simulink model "MPC_FL_CBFcontroller"  (R2026a)
settings: Solver=VariableStepAuto  StopTime=120
PreLoadFcn:
  | % Define variants
  | VSS_PATH_CTRL_PURE_PURSUIT=Simulink.Variant('VSS_PATH_CTRL_MODE==1');
  | VSS_PATH_CTRL_REAR_WHEEL=Simulink.Variant('VSS_PATH_CTRL_MODE==2');
  | % Select default variant
  | VSS_PATH_CTRL_MODE =1;
  | 
  | 
  | % Longitudinal PID
  | LongitudinalPID.Kp = 20;
  | LongitudinalPID.Ki = 0;
  | LongitudinalPID.Kd = 0;
  | LongitudinalPID.N = 100;
  | LongitudinalPID.MaxAccel = 80;
  | LongitudinalPID.SampleTime = 0.01;
  | 
  | % Steering PID
  | SteeringPID.Kp = 60;
  | SteeringPID.Ki = 0;
  | SteeringPID.Kd = 5;
  | SteeringPID.N = 10;
  | SteeringPID.MaxSpeed =  10;
  | SteeringPID.MinSpeed = -10;
  | SteeringPID.SampleTime = 0.01;
  | 
  | 
  | 
  | setSMVehicleVisuParameters;
  | 
  | % Load planner commands
  | load('PlannerCmdTests.mat');
  | % Assign one for testing:
  | plannerCmd = plannerCmdFwd;
  | % plannerCmd  = plannerCmdFwdBwd;
  | 
  | % Bus structure definition
  | load('PlannerBusStruct.mat');
  | 
  | % Rear Wheel Controller Parameters
  | RW.k_e = 0.2;    % 0.1
  | RW.k_theta = 1;   % 0.75
  | RW.SampleTime =  0.1;
  | RW.GoalRadius = 0.3;
  | 
  | % Pure pursuit parameters
  | PP.DesiredLinearVel = 5;
  | PP.MaxAngularVel  = 10;
  | PP.LookaheadDist  = 1;
  | PP.Wheelbase = 4;
  | PP.GoalRadius = 0.1;
  | PP.SampleTime = 0.1;
  | PP.LongitudinalPID.Kp = 20;
  | PP.LongitudinalPID.Ki = 0;
  | PP.LongitudinalPID.Kd = 0;
  | PP.LongitudinalPID.N = 100;
  | PP.LongitudinalPID.MaxLongAccel =  80;
  | PP.LongitudinalPID.MinLongAccel = -80;
  | 
  | % Spline ref
  | splineRef = [ 0 0 0;[plannerCmd.PathMatrix(1:plannerCmd.PathLengths(1),1:2,1),0*ones(length(plannerCmd.PathMatrix(1:plannerCmd.PathLengths(1),1,1)),1)]];
values from neighbouring files (symbols this model uses):
  m = max(2, ceil(Lseg/ds))    [Trajectory.m]    (also in plot_nmpc_result.m = NaN)
  s = [0; cumsum(hypot(diff(xs),diff(ys)))]    [Trajectory.m]    (also in plot_parking_mpc.m = evalin('base',name); plot_result.m = out.(names{k}))
  trajMatrix = [tvec, xd, yd, thd, vd, wd]    [Trajectory.m]    (also in plot_parking_mpc.m = evalin('base','trajMatrix'); plot_result.m = evalin('base','trajMatrix'))
undefined symbols (not defined in the file or in its folder): DiscIntNeverNeededParam, smvv, X, Y, Z
libraries: sm_lib x527, sm_vehicle_slalom_lib x48, fl_lib x40, fl_ps_legacy_lib x28, nesl_utility x13
(part 15 of 15)

== system MPC_FL_CBFcontroller/Robot Bicycle Model/Visualizer/SM_Car_Visu/Vehicle7/Steering_Wheel/Logo/LStick3 ==
  Stick : sm_lib/Body Elements/Brick Solid  BrickDimensions=[smvv.steeringwheel.letterStick 0.001 0.001]  BrickDimensionsUnits=m  ExportEntireGeometry=off  InertiaType=PointMass  BasedOnType=Density  Density=1000  DensityUnits=kg/m^3  Mass=0.001  MassUnits=kg  CenterOfMass=[0 0 0]  CenterOfMassUnits=m  MomentsOfInertia=[1 1 1]  MomentsOfInertiaUnits=kg*m^2  ProductsOfInertia=[1 1 1]  ProductsOfInertiaUnits=kg*m^2  GraphicType=FromGeometry  MarkerShape=Sphere  MarkerSize=10  GraphicVisPropType=SimpleVisualProperties  GraphicDiffuseColor=smvv.steeringwheel.letterColor  GraphicOpacity=1.0  GraphicSpecularColor=[0.5 0.5 0.5 1.0]  GraphicAmbientColor=[0.15 0.15 0.15 1.0]  GraphicEmissiveColor=[0.0 0.0 0.0 1.0]  GraphicShininess=75  DoExposeReferenceFrame=on  SerializedFrames=<Frames/>
  X offset 1 : sm_lib/Frames and Transforms/Rigid Transform  RotationMethod=None  FollAlignAxisA=+X  BaseAlignAxisA=+Y  FollAlignAxisB=+Y  BaseAlignAxisB=+Z  RotationStandardAxis=+X  RotationAngle=0  RotationAngleUnits=deg  RotationArbitraryAxis=[0 0 1]  RotationSequenceAxes=FollowerAxes  RotationSequence=XYX  RotationSequenceAngles=[0 0 0]  RotationSequenceAnglesUnits=deg  RotationMatrix=[1 0 0; 0 1 0; 0 0 1]  Quaternion=[1 0 0 0]  TranslationMethod=StandardAxis  TranslationCartesianOffset=[0 0 0]  TranslationCartesianOffsetUnits=m  TranslationStandardAxis=-X  TranslationStandardOffset=0.5*smvv.steeringwheel.letterStick  TranslationStandardOffsetUnits=m  TranslationROffset=0  TranslationROffsetUnits=m  TranslationThetaOffset=0  TranslationThetaOffsetUnits=deg  TranslationZOffset=0  TranslationZOffsetUnits=m
  x offset 2 : sm_lib/Frames and Transforms/Rigid Transform  RotationMethod=None  FollAlignAxisA=+X  BaseAlignAxisA=+Y  FollAlignAxisB=+Y  BaseAlignAxisB=+Z  RotationStandardAxis=+X  RotationAngle=0  RotationAngleUnits=deg  RotationArbitraryAxis=[0 0 1]  RotationSequenceAxes=FollowerAxes  RotationSequence=XYX  RotationSequenceAngles=[0 0 0]  RotationSequenceAnglesUnits=deg  RotationMatrix=[1 0 0; 0 1 0; 0 0 1]  Quaternion=[1 0 0 0]  TranslationMethod=StandardAxis  TranslationCartesianOffset=[0 0 0]  TranslationCartesianOffsetUnits=m  TranslationStandardAxis=+X  TranslationStandardOffset=0.5*smvv.steeringwheel.letterStick  TranslationStandardOffsetUnits=m  TranslationROffset=0  TranslationROffsetUnits=m  TranslationThetaOffset=0  TranslationThetaOffsetUnits=deg  TranslationZOffset=0  TranslationZOffsetUnits=m
  Conn1 : PMIOPort  Side=Left
  Conn2 : PMIOPort  Port=2  Side=Right
  connections:
  X offset 1/RConn1 -- Conn1/RConn1
  x offset 2/RConn1 -- Conn2/RConn1
  x offset 2/LConn1 -- Stick/RConn1 -- X offset 1/LConn1

== system MPC_FL_CBFcontroller/Robot Bicycle Model/Visualizer/SM_Car_Visu/Vehicle7/Steering_Wheel/Logo/LStick4 ==
  Stick : sm_lib/Body Elements/Brick Solid  BrickDimensions=[smvv.steeringwheel.letterStick 0.001 0.001]  BrickDimensionsUnits=m  ExportEntireGeometry=off  InertiaType=PointMass  BasedOnType=Density  Density=1000  DensityUnits=kg/m^3  Mass=0.001  MassUnits=kg  CenterOfMass=[0 0 0]  CenterOfMassUnits=m  MomentsOfInertia=[1 1 1]  MomentsOfInertiaUnits=kg*m^2  ProductsOfInertia=[1 1 1]  ProductsOfInertiaUnits=kg*m^2  GraphicType=FromGeometry  MarkerShape=Sphere  MarkerSize=10  GraphicVisPropType=SimpleVisualProperties  GraphicDiffuseColor=smvv.steeringwheel.letterColor  GraphicOpacity=1.0  GraphicSpecularColor=[0.5 0.5 0.5 1.0]  GraphicAmbientColor=[0.15 0.15 0.15 1.0]  GraphicEmissiveColor=[0.0 0.0 0.0 1.0]  GraphicShininess=75  DoExposeReferenceFrame=on  SerializedFrames=<Frames/>
  X offset 1 : sm_lib/Frames and Transforms/Rigid Transform  RotationMethod=None  FollAlignAxisA=+X  BaseAlignAxisA=+Y  FollAlignAxisB=+Y  BaseAlignAxisB=+Z  RotationStandardAxis=+X  RotationAngle=0  RotationAngleUnits=deg  RotationArbitraryAxis=[0 0 1]  RotationSequenceAxes=FollowerAxes  RotationSequence=XYX  RotationSequenceAngles=[0 0 0]  RotationSequenceAnglesUnits=deg  RotationMatrix=[1 0 0; 0 1 0; 0 0 1]  Quaternion=[1 0 0 0]  TranslationMethod=StandardAxis  TranslationCartesianOffset=[0 0 0]  TranslationCartesianOffsetUnits=m  TranslationStandardAxis=-X  TranslationStandardOffset=0.5*smvv.steeringwheel.letterStick  TranslationStandardOffsetUnits=m  TranslationROffset=0  TranslationROffsetUnits=m  TranslationThetaOffset=0  TranslationThetaOffsetUnits=deg  TranslationZOffset=0  TranslationZOffsetUnits=m
  Conn1 : PMIOPort  Side=Left
  connections:
  Stick/RConn1 -- X offset 1/LConn1
  X offset 1/RConn1 -- Conn1/RConn1

== system MPC_FL_CBFcontroller/Robot Bicycle Model/Visualizer/SM_Car_Visu/Vehicle7/Steering_Wheel/Logo/LStick5 ==
  Stick : sm_lib/Body Elements/Brick Solid  BrickDimensions=[smvv.steeringwheel.letterStick 0.001 0.001]  BrickDimensionsUnits=m  ExportEntireGeometry=off  InertiaType=PointMass  BasedOnType=Density  Density=1000  DensityUnits=kg/m^3  Mass=0.001  MassUnits=kg  CenterOfMass=[0 0 0]  CenterOfMassUnits=m  MomentsOfInertia=[1 1 1]  MomentsOfInertiaUnits=kg*m^2  ProductsOfInertia=[1 1 1]  ProductsOfInertiaUnits=kg*m^2  GraphicType=FromGeometry  MarkerShape=Sphere  MarkerSize=10  GraphicVisPropType=SimpleVisualProperties  GraphicDiffuseColor=smvv.steeringwheel.letterColor  GraphicOpacity=1.0  GraphicSpecularColor=[0.5 0.5 0.5 1.0]  GraphicAmbientColor=[0.15 0.15 0.15 1.0]  GraphicEmissiveColor=[0.0 0.0 0.0 1.0]  GraphicShininess=75  DoExposeReferenceFrame=on  SerializedFrames=<Frames/>
  X offset 1 : sm_lib/Frames and Transforms/Rigid Transform  RotationMethod=None  FollAlignAxisA=+X  BaseAlignAxisA=+Y  FollAlignAxisB=+Y  BaseAlignAxisB=+Z  RotationStandardAxis=+X  RotationAngle=0  RotationAngleUnits=deg  RotationArbitraryAxis=[0 0 1]  RotationSequenceAxes=FollowerAxes  RotationSequence=XYX  RotationSequenceAngles=[0 0 0]  RotationSequenceAnglesUnits=deg  RotationMatrix=[1 0 0; 0 1 0; 0 0 1]  Quaternion=[1 0 0 0]  TranslationMethod=StandardAxis  TranslationCartesianOffset=[0 0 0]  TranslationCartesianOffsetUnits=m  TranslationStandardAxis=-X  TranslationStandardOffset=0.5*smvv.steeringwheel.letterStick  TranslationStandardOffsetUnits=m  TranslationROffset=0  TranslationROffsetUnits=m  TranslationThetaOffset=0  TranslationThetaOffsetUnits=deg  TranslationZOffset=0  TranslationZOffsetUnits=m
  x offset 2 : sm_lib/Frames and Transforms/Rigid Transform  RotationMethod=None  FollAlignAxisA=+X  BaseAlignAxisA=+Y  FollAlignAxisB=+Y  BaseAlignAxisB=+Z  RotationStandardAxis=+X  RotationAngle=0  RotationAngleUnits=deg  RotationArbitraryAxis=[0 0 1]  RotationSequenceAxes=FollowerAxes  RotationSequence=XYX  RotationSequenceAngles=[0 0 0]  RotationSequenceAnglesUnits=deg  RotationMatrix=[1 0 0; 0 1 0; 0 0 1]  Quaternion=[1 0 0 0]  TranslationMethod=StandardAxis  TranslationCartesianOffset=[0 0 0]  TranslationCartesianOffsetUnits=m  TranslationStandardAxis=+X  TranslationStandardOffset=0.5*smvv.steeringwheel.letterStick  TranslationStandardOffsetUnits=m  TranslationROffset=0  TranslationROffsetUnits=m  TranslationThetaOffset=0  TranslationThetaOffsetUnits=deg  TranslationZOffset=0  TranslationZOffsetUnits=m
  Conn1 : PMIOPort  Side=Left
  Conn2 : PMIOPort  Port=2  Side=Right
  connections:
  X offset 1/RConn1 -- Conn1/RConn1
  x offset 2/RConn1 -- Conn2/RConn1
  x offset 2/LConn1 -- Stick/RConn1 -- X offset 1/LConn1

== system MPC_FL_CBFcontroller/Robot Bicycle Model/Visualizer/SM_Car_Visu/Vehicle7/Steering_Wheel/Logo/LStick6 ==
  Stick : sm_lib/Body Elements/Brick Solid  BrickDimensions=[2*smvv.steeringwheel.letterStick 0.001 0.001]  BrickDimensionsUnits=m  ExportEntireGeometry=off  InertiaType=PointMass  BasedOnType=Density  Density=1000  DensityUnits=kg/m^3  Mass=0.001  MassUnits=kg  CenterOfMass=[0 0 0]  CenterOfMassUnits=m  MomentsOfInertia=[1 1 1]  MomentsOfInertiaUnits=kg*m^2  ProductsOfInertia=[1 1 1]  ProductsOfInertiaUnits=kg*m^2  GraphicType=FromGeometry  MarkerShape=Sphere  MarkerSize=10  GraphicVisPropType=SimpleVisualProperties  GraphicDiffuseColor=smvv.steeringwheel.letterColor  GraphicOpacity=1.0  GraphicSpecularColor=[0.5 0.5 0.5 1.0]  GraphicAmbientColor=[0.15 0.15 0.15 1.0]  GraphicEmissiveColor=[0.0 0.0 0.0 1.0]  GraphicShininess=75  DoExposeReferenceFrame=on  SerializedFrames=<Frames/>
  X offset 1 : sm_lib/Frames and Transforms/Rigid Transform  RotationMethod=None  FollAlignAxisA=+X  BaseAlignAxisA=+Y  FollAlignAxisB=+Y  BaseAlignAxisB=+Z  RotationStandardAxis=+X  RotationAngle=0  RotationAngleUnits=deg  RotationArbitraryAxis=[0 0 1]  RotationSequenceAxes=FollowerAxes  RotationSequence=XYX  RotationSequenceAngles=[0 0 0]  RotationSequenceAnglesUnits=deg  RotationMatrix=[1 0 0; 0 1 0; 0 0 1]  Quaternion=[1 0 0 0]  TranslationMethod=StandardAxis  TranslationCartesianOffset=[0 0 0]  TranslationCartesianOffsetUnits=m  TranslationStandardAxis=-X  TranslationStandardOffset=smvv.steeringwheel.letterStick  TranslationStandardOffsetUnits=m  TranslationROffset=0  TranslationROffsetUnits=m  TranslationThetaOffset=0  TranslationThetaOffsetUnits=deg  TranslationZOffset=0  TranslationZOffsetUnits=m
  x offset 2 : sm_lib/Frames and Transforms/Rigid Transform  RotationMethod=None  FollAlignAxisA=+X  BaseAlignAxisA=+Y  FollAlignAxisB=+Y  BaseAlignAxisB=+Z  RotationStandardAxis=+X  RotationAngle=0  RotationAngleUnits=deg  RotationArbitraryAxis=[0 0 1]  RotationSequenceAxes=FollowerAxes  RotationSequence=XYX  RotationSequenceAngles=[0 0 0]  RotationSequenceAnglesUnits=deg  RotationMatrix=[1 0 0; 0 1 0; 0 0 1]  Quaternion=[1 0 0 0]  TranslationMethod=StandardAxis  TranslationCartesianOffset=[0 0 0]  TranslationCartesianOffsetUnits=m  TranslationStandardAxis=+X  TranslationStandardOffset=smvv.steeringwheel.letterStick  TranslationStandardOffsetUnits=m  TranslationROffset=0  TranslationROffsetUnits=m  TranslationThetaOffset=0  TranslationThetaOffsetUnits=deg  TranslationZOffset=0  TranslationZOffsetUnits=m
  Conn1 : PMIOPort  Side=Left
  Conn2 : PMIOPort  Port=2  Side=Right
  connections:
  X offset 1/LConn1 -- Stick/RConn1 -- x offset 2/LConn1
  x offset 2/RConn1 -- Conn2/RConn1
  X offset 1/RConn1 -- Conn1/RConn1

== system MPC_FL_CBFcontroller/Robot Bicycle Model/Visualizer/SM_Car_Visu/Vehicle7/Steering_Wheel/Logo/LStick7 ==
  Stick : sm_lib/Body Elements/Brick Solid  BrickDimensions=[smvv.steeringwheel.letterStick 0.001 0.001]  BrickDimensionsUnits=m  ExportEntireGeometry=off  InertiaType=PointMass  BasedOnType=Density  Density=1000  DensityUnits=kg/m^3  Mass=0.001  MassUnits=kg  CenterOfMass=[0 0 0]  CenterOfMassUnits=m  MomentsOfInertia=[1 1 1]  MomentsOfInertiaUnits=kg*m^2  ProductsOfInertia=[1 1 1]  ProductsOfInertiaUnits=kg*m^2  GraphicType=FromGeometry  MarkerShape=Sphere  MarkerSize=10  GraphicVisPropType=SimpleVisualProperties  GraphicDiffuseColor=smvv.steeringwheel.letterColor  GraphicOpacity=1.0  GraphicSpecularColor=[0.5 0.5 0.5 1.0]  GraphicAmbientColor=[0.15 0.15 0.15 1.0]  GraphicEmissiveColor=[0.0 0.0 0.0 1.0]  GraphicShininess=75  DoExposeReferenceFrame=on  SerializedFrames=<Frames/>
  X offset 1 : sm_lib/Frames and Transforms/Rigid Transform  RotationMethod=None  FollAlignAxisA=+X  BaseAlignAxisA=+Y  FollAlignAxisB=+Y  BaseAlignAxisB=+Z  RotationStandardAxis=+X  RotationAngle=0  RotationAngleUnits=deg  RotationArbitraryAxis=[0 0 1]  RotationSequenceAxes=FollowerAxes  RotationSequence=XYX  RotationSequenceAngles=[0 0 0]  RotationSequenceAnglesUnits=deg  RotationMatrix=[1 0 0; 0 1 0; 0 0 1]  Quaternion=[1 0 0 0]  TranslationMethod=StandardAxis  TranslationCartesianOffset=[0 0 0]  TranslationCartesianOffsetUnits=m  TranslationStandardAxis=-X  TranslationStandardOffset=0.5*smvv.steeringwheel.letterStick  TranslationStandardOffsetUnits=m  TranslationROffset=0  TranslationROffsetUnits=m  TranslationThetaOffset=0  TranslationThetaOffsetUnits=deg  TranslationZOffset=0  TranslationZOffsetUnits=m
  Conn1 : PMIOPort  Side=Left
  connections:
  X offset 1/RConn1 -- Conn1/RConn1
  Stick/RConn1 -- X offset 1/LConn1

== matlab function MPC_FL_CBFcontroller/MATLAB Function1 ==
  data: pose input; v_out output; u1_cmd input; u2_cmd input; delta_out output; h_min_out output; qp_status output; h_red_out output; h_pink_out output; h_obs3_out output
function [v_out, delta_out, h_min_out, qp_status, ...
          h_red_out, h_pink_out, h_obs3_out] = ...
    fl_cbf_inner_filter_u1u2_reverse(pose, u1_cmd, u2_cmd)
% Fast feedback-linearization + CBF safety filter for the reverse-phase outer.
%
% Inputs u1_cmd and u2_cmd are the virtual velocity of the point
%   P = [x;y] + ell*[cos(theta);sin(theta)].
% This block converts them to q = [v; v*tan(delta)] and projects q into
% the CBF-safe and actuator-limited set.

coder.extrinsic('quadprog');
coder.extrinsic('optimoptions');

%% Parameters
% IMPORTANT: set this equal to the sample time of this MATLAB Function
% block. For a 100 Hz inner loop use 0.01; for 50 Hz use 0.02.
Ts = 0.01;

L        = 3.0;
ell      = L;
vMin     = -2.5;
vMax     =  3.0;
dMax     = 60*pi/180;
tanDMax  = tan(dMax);
aMax     = 3.0;
dRate    = 0.60;
gammaCBF = 0.30;

% Obstacle circles: [cx, cy, inflated radius].
obs = [53.5, 21.0, 3.64;   % red, rear  (unchanged)
    56.5, 21.0, 3.64;   % red, front (unchanged)
    37.5, 21.0, 3.64;   % pink, rear  ← FIX: was 38.5, should be 37.5
    40.5, 21.0, 3.64;   % pink, front (correct)
    26.6, 17.0, 3.24];  % obstacle 3  (unchanged)

nObs = 5;

%% Persistent actuator state and gear hysteresis
persistent prevV prevDelta gear

if isempty(prevV) || isempty(prevDelta) || isempty(gear)
    prevV     = 0.0;
    prevDelta = 0.0;
    gear      = 1.0;
end

pose = double(pose(:));
pose = pose(1:3);
pose(3) = atan2(sin(pose(3)),cos(pose(3)));

uRef = [double(u1_cmd);double(u2_cmd)];

th = pose(3);
eTheta = [cos(th);sin(th)];
ePerp  = [-sin(th);cos(th)];

% P_dot = eTheta*v + (ell/L)*ePerp*(v*tan(delta)).
% Therefore:
%   v          = eTheta.'*uRef
%   v*tan(del) = (L/ell)*ePerp.'*uRef
vNom  = eTheta.'*uRef;
q2Nom = (L/ell)*(ePerp.'*uRef);
vNom  = max(vMin,min(vMax,vNom));

% Gear hysteresis prevents rapid switching between forward and reverse
% steering cones when the planned longitudinal velocity crosses zero.
if gear >= 0.0
    if vNom < -0.15
        gear = -1.0;
    end
else
    if vNom > 0.15
        gear = 1.0;
    end
end

if abs(vNom) <= 0.15 && abs(prevV) > 0.20
    gear = sign(prevV);
end

%% Current barrier diagnostics
hRedOut = minimumBarrierAgainstSet(pose,obs(1:2,:),L);
hPinkOut = minimumBarrierAgainstSet(pose,obs(3:4,:),L);
hObs3Out = minimumBarrierAgainstSet(pose,obs(5:5,:),L);

h_red_out  = hRedOut;
h_pink_out = hPinkOut;
h_obs3_out = hObs3Out;
h_min_out  = min(hRedOut,min(hPinkOut,hObs3Out));

%% Nominal auxiliary input obtained from feedback linearization
qNom = [vNom;q2Nom];

% Penalize changes in velocity more than changes in the auxiliary steering
% variable. The exact steering wheel is recovered after the QP.
wV = 8.0;
wQ = 2.0;

H = diag([2.0*wV,2.0*wQ]);
f = [-2.0*wV*qNom(1);
     -2.0*wQ*qNom(2)];

% Suppress repeated solver messages in the Simulation Diagnostics window.
qpOptions = optimoptions('quadprog', ...
    'Algorithm','interior-point-convex','Display','off');

%% Bounds and actuator-rate limits
dvMax = aMax*Ts;
ddMax = dRate*Ts;

q2Prev = prevV*tan(prevDelta);

% This box is a conservative linear approximation of steering-rate
% limiting in q-space.
dq2Max = abs(prevV)*ddMax + dvMax*tanDMax + 0.02;

lb = [max(vMin,prevV-dvMax);
      max(-vMax*tanDMax,q2Prev-dq2Max)];

ub = [min(vMax,prevV+dvMax);
      min( vMax*tanDMax,q2Prev+dq2Max)];

%% Try the selected gear cone first, then the opposite cone if necessary
qSol       = [0.0;0.0];
exitStatus = -100.0;
solved     = false;
usedGear   = gear;

for attempt = 1:2
    if attempt == 1
        gearTry = gear;
    else
        gearTry = -gear;
    end

    Aineq = zeros(2*nObs+2,2);
    bineq = zeros(2*nObs+2,1);
    row = 0;

    % Exact sufficient linear DCBF constraints for both ego circles.
    for j = 1:nObs
        cx = obs(j,1);
        cy = obs(j,2);
        rr = obs(j,3);

        [hRear,aRear] = rearCbfRow(pose,cx,cy,rr,Ts);
        row = row+1;
        Aineq(row,:) = aRear.';
        bineq(row)   = gammaCBF*hRear;

        [hFront,aFront] = frontCbfRow(pose,cx,cy,rr,Ts,L);
        row = row+1;
        Aineq(row,:) = aFront.';
        bineq(row)   = gammaCBF*hFront;
    end

    % Steering cone. Because q2=v*tan(delta), the feasible steering cone
    % depends on the direction of motion.
    if gearTry >= 0.0
        % Forward: |q2| <= tan(dMax)*q1. This also enforces q1 >= 0.
        row = row+1;
        Aineq(row,:) = [-tanDMax,  1.0];
        bineq(row)   = 0.0;

        row = row+1;
        Aineq(row,:) = [-tanDMax, -1.0];
        bineq(row)   = 0.0;
    else
        % Reverse: tan(dMax)*q1 <= q2 <= -tan(dMax)*q1.
        % This also enforces q1 <= 0.
        row = row+1;
        Aineq(row,:) = [tanDMax,  1.0];
        bineq(row)   = 0.0;

        row = row+1;
        Aineq(row,:) = [tanDMax, -1.0];
        bineq(row)   = 0.0;
    end

    % quadprog returns an empty q when it declares the QP infeasible.
    % Keep the raw output variable-size and copy only after checking its
    % length, preventing a 2x1 versus 0x0 runtime mismatch.
    qTryRaw = zeros(0,1);
    coder.varsize('qTryRaw',[2 1],[true false]);
    exitTry = 0.0;

    [qTryRaw,~,exitTry] = quadprog( ...
        H,f,Aineq,bineq,[],[],lb,ub,[],qpOptions);

    qTry = zeros(2,1);
    qTryOK = false;

    if exitTry > 0 && size(qTryRaw,1) == 2
        qTry(:) = qTryRaw(1:2);
        qTryOK = true;

        if ~isfinite(qTry(1)) || ~isfinite(qTry(2))
            qTryOK = false;
        end
    end

    if qTryOK
        qSol       = qTry;
        exitStatus = exitTry;
        solved     = true;
        usedGear   = gearTry;
        break;
    end
end

%% Convert auxiliary input to actuator commands
if solved
    vOut = qSol(1);

    if abs(vOut) < 1e-4
        vOut     = 0.0;
        deltaOut = prevDelta;
    else
        deltaOut = atan(qSol(2)/vOut);
    end

    vOut     = max(vMin,min(vMax,vOut));
    deltaOut = max(-dMax,min(dMax,deltaOut));

    % Keep the persistent cone consistent with the successful QP cone.
    gear = usedGear;
else
    % If both cones are infeasible, stop. If the current state is safe,
    % zero velocity keeps the one-step state inside the safe set.
    vOut       = 0.0;
    deltaOut   = prevDelta;
    exitStatus = -10.0;
end

v_out     = vOut;
delta_out = deltaOut;
qp_status = exitStatus;

prevV     = v_out;
prevDelta = delta_out;

end

%% -----------------------------------------------------------------------
function hMin = minimumBarrierAgainstSet(x,obsSet,L)

nLocal = size(obsSet,1);
hMin = 1.0e12;

for j = 1:nLocal
    cx = obsSet(j,1);
    cy = obsSet(j,2);
    rr = obsSet(j,3);

    hRear = rearBarrier(x,cx,cy,rr);
    hFront = frontBarrier(x,cx,cy,rr,L);
    hBoth = min(hRear,hFront);

    if hBoth < hMin
        hMin = hBoth;
    end
end

end

%% -----------------------------------------------------------------------
function h = rearBarrier(x,cx,cy,r)

dx = x(1)-cx;
dy = x(2)-cy;
h  = dx*dx+dy*dy-r*r;

end

%% -----------------------------------------------------------------------
function h = frontBarrier(x,cx,cy,r,L)

th = x(3);
px = x(1)+L*cos(th);
py = x(2)+L*sin(th);

dx = px-cx;
dy = py-cy;
h  = dx*dx+dy*dy-r*r;

end

%% -----------------------------------------------------------------------
function [h,a] = rearCbfRow(x,cx,cy,r,Ts)
% Rear ego center moves as p_next = p + Ts*e*q1.
% h_next = h + 2*d'*G*q + ||G*q||^2, so
% 2*d'*G*q >= -gamma*h is sufficient for h_next >= (1-gamma)*h.

th = x(3);
e = [cos(th);sin(th)];

d = [x(1)-cx;
     x(2)-cy];

h = d.'*d-r*r;

G = [Ts*e, zeros(2,1)];

% We need 2*d'*G*q >= -gamma*h, i.e. -2*d'*G*q <= gamma*h.
a = -2.0*(d.'*G).';

end

%% -----------------------------------------------------------------------
function [h,a] = frontCbfRow(x,cx,cy,r,Ts,L)
% Front ego center moves as
% p_next = p + Ts*e*q1 + Ts*e_perp*q2,
% where q2 = v*tan(delta).

th = x(3);
e     = [cos(th);sin(th)];
ePerp = [-sin(th);cos(th)];

px = x(1)+L*cos(th);
py = x(2)+L*sin(th);

d = [px-cx;
     py-cy];

h = d.'*d-r*r;

G = Ts*[e,ePerp];

a = -2.0*(d.'*G).';

end

== matlab function MPC_FL_CBFcontroller/MATLAB Function ==
  data: pose input; trajectory input; u1_cmd output; t input; u2_cmd output; P_pred_out output; qp_status output; scp_passes_out output; mode_out output
function [u1_cmd, u2_cmd, P_pred_out, qp_status, scp_passes_out, mode_out] = ...
    mpc_outer_linear_cbf_reverse(pose, trajectory, t)
% Updated outer MPC-CBF for the feedback-linearized vehicle point P.
%
% Inputs:
%   pose       = [x_rear; y_rear; theta]
%   trajectory = [t, x_rear, y_rear, theta, v, kappa]
%   t          = current simulation time
%
% Outputs:
%   u1_cmd,u2_cmd  virtual velocity of the feedback-linearized point P
%   P_pred_out     2 x (Np+1) predicted positions of P
%   qp_status      status of the last successful QP
%   scp_passes_out number of successful SCP passes
%   mode_out       1=TRACK, 2=AVOID, 3=REJOIN, 4=STOP AT S-START,
%                    5=REVERSE-S, 6=PARKED
%
% Important:
%   This version preserves the u1/u2 feedback-linearized architecture.
%   The inner block must convert [u1;u2] to [v;delta] using the same
%   feedback-linearization distance ell = L.

coder.extrinsic('quadprog');
coder.extrinsic('optimoptions');

%% User parameters
Ts   = 0.20;
Np   = 5;
nSCP = 3;

L   = 3.0;
ell = L;

uMax = 3.0;

Q     = 20.0*eye(2);
Qf    = 80.0*eye(2);
R     = 0.40*eye(2);
rhoDu = 1.20;

gammaCBF = 0.3;
scpTrust = 1.25;

%% Vehicle and obstacle parameters
rVeh        = 1.6;
carHalfSpace = 1.5;
marginOuter = 0.4 + 0.05*0.8;
marginInner = marginOuter;

% Conservative single-circle model around the feedback-linearized point P.
% For either parked car:
%   parked-car envelope = 1.5 + 1.6 = 3.1 m
%   ego envelope around P = ell + 1.6 = 3.1 m
%   total separation      = 3.1 + 3.1 + 0.44 = 6.64 m
% Reduced outer planning radius. The inner two-circle CBF remains the
% exact hard safety layer, so the outer single circle need not carry the
% full midpoint-envelope inflation.
rOuterCar = 4.20;

% Obstacle 3 has physical radius 1.2 m.
rObs3   = 1.2;
% Slightly larger than the exact inner separation of 3.24 m, but much
% less conservative than the full midpoint-envelope value of 4.74 m.
rOuter3 = 3.30;

% Exact two-ego-circle separation used for mode-exit diagnostics.
rPair3 = rObs3+rVeh+marginInner;

% [cx, cy, outer-MPC radius]
obs = [55.0, 21.0, rOuterCar;   % red parked car
       39.0, 21.0, rOuterCar;   % pink parked car
       26.6, 17.0, rOuter3];    % obstacle 3

nObs = 3;

xObs3 = obs(3,1);
yObs3 = obs(3,2);

% Rear-axle progress gates. The corresponding P gates are obtained by
% shifting ell forward because the gate heading is approximately zero.
gateRear1 = [21.0;13.0];
gateRear2 = [31.0;13.0];
gateTheta = 0.0;

% Explicit reverse-parking phase gates.
yLane       = 16.36;
reverseRear = [60.0;yLane];
xGoal = (55.0 + 39.0)/2 - L/2 - 1.0; 
goalRear    = [xGoal;21.0];
tReverseStart = findReverseStartTime(trajectory);

%% Persistent data
nInputs = 2*Np;
nz      = nInputs+1;    % last variable is the CBF slack

persistent zWarm uPrev tPrev mode refOffset avoidPhase

if isempty(zWarm) || isempty(uPrev) || isempty(tPrev) || ...
        isempty(mode) || isempty(refOffset) || isempty(avoidPhase)
    zWarm      = zeros(nz,1);
    uPrev      = zeros(2,1);
    tPrev      = t;
    mode       = 1.0;
    refOffset  = 0.0;
    avoidPhase = 1.0;
end

% Detect a simulation restart.
if t < tPrev - 1e-9
    zWarm      = zeros(nz,1);
    uPrev      = zeros(2,1);
    mode       = 1.0;
    refOffset  = 0.0;
    avoidPhase = 1.0;
end

pose = double(pose(:));
pose = pose(1:3);
pose(3) = atan2(sin(pose(3)),cos(pose(3)));

ct = cos(pose(3));
st = sin(pose(3));

p0 = [pose(1)+ell*ct;
      pose(2)+ell*st];

%% Hybrid mode logic
oldMode = mode;

% Exact current barrier to obstacle 3, using both ego circles.
hObs3Now = obstacle3Barrier(pose,xObs3,yObs3,rPair3,L);
distanceAhead3 = xObs3-pose(1);

if mode == 1.0
    % Start the lower bypass before the vehicle becomes head-on at the
    % obstacle boundary.
    if distanceAhead3 > 0.0 && distanceAhead3 < 20.0 && ...
            abs(pose(2)-yObs3) < 6.0
        mode       = 2.0;
        avoidPhase = 1.0;
    end

elseif mode == 2.0
    % First reach the safe pre-obstacle gate, then target the
    % post-obstacle gate. This explicitly selects the lower side and
    % prevents the nonconvex SCP from settling into the braking solution.
    if avoidPhase == 1.0
        distGate1 = hypot(pose(1)-gateRear1(1), ...
                          pose(2)-gateRear1(2));

        if distGate1 < 0.8 || ...
                (pose(1) > gateRear1(1)+1.0 && pose(2) < 13.2)
            avoidPhase = 2.0;
            zWarm(:)   = 0.0;
        end
    end

    % Rejoin only after the vehicle has passed obstacle 3 with positive
    % exact two-circle clearance.
    if pose(1) > gateRear2(1) && hObs3Now > 0.50
        mode       = 3.0;
        avoidPhase = 1.0;

        % Re-anchor the timed reference at the current forward x-position.
        rejoinRefTime = findReferenceTimeAtX(trajectory,pose(1));
        refOffset     = rejoinRefTime-t;
    end

elseif mode == 3.0
    tRefNow = t+refOffset;
    [xrNow,yrNow,thrNow,~,~] = interpolateReference(trajectory,tRefNow);

    posError = hypot(pose(1)-xrNow,pose(2)-yrNow);
    thError  = atan2(sin(pose(3)-thrNow),cos(pose(3)-thrNow));

    if posError < 0.35 && abs(thError) < 0.20 && hObs3Now > 0.50
        mode = 1.0;
    end

elseif mode == 4.0
    % Wait until the vehicle is stopped at the reverse-S start pose.
    % uPrev is the previous virtual velocity command and is used as a
    % practical outer-loop velocity estimate.
    distReverseStart = hypot(pose(1)-reverseRear(1), ...
                             pose(2)-reverseRear(2));
    outerSpeed = norm(uPrev);

    if distReverseStart < 0.25 && abs(pose(3)) < 0.15 && ...
            outerSpeed < 0.10
        mode      = 5.0;
        refOffset = tReverseStart-t;
    end

elseif mode == 5.0
    % Reverse-S phase: track the timed reference beginning exactly at its
    % first negative-v sample. The red/pink CBF constraints remain active.
    distGoal = hypot(pose(1)-goalRear(1),pose(2)-goalRear(2));

    if distGoal < 0.25 && norm(uPrev) < 0.10
        mode = 6.0;
    end

elseif mode == 6.0
    % Parked: hold the goal pose.
    mode = 6.0;
end

% Do not let the timed forward reference run into the reverse-S section
% while the actual vehicle is still approaching x=60. Switch to a dedicated
% stop-at-reverse-start mode first.
if (mode == 1.0 || mode == 3.0) && pose(1) > 56.0
    mode = 4.0;
end

if mode ~= oldMode
    zWarm(:) = 0.0;
end

mode_out = mode;
tRef = t+refOffset;

%% Construct the position and virtual-input references
ref = trajectory;

Pref = zeros(2,Np);
Uref = zeros(2,Np);

if mode == 2.0
    if avoidPhase == 1.0
        gateRear = gateRear1;
    else
        gateRear = gateRear2;
    end

    gateP = [gateRear(1)+ell*cos(gateTheta);
             gateRear(2)+ell*sin(gateTheta)];

    % Straight-line supervisory target only. The QP and CBF constraints
    % generate the actual online trajectory between the gates.
    uGate = (gateP-p0)/(Np*Ts);

    for i = 1:2
        uGate(i) = max(-uMax,min(uMax,uGate(i)));
    end

    for k = 1:Np
        alpha = k/Np;
        Pref(:,k) = (1.0-alpha)*p0+alpha*gateP;
        Uref(:,k) = uGate;
    end

elseif mode == 4.0
    % Stop at the reverse-S start pose. This prevents the timed reference
    % from entering the reverse segment before the vehicle is ready.
    reverseP = [reverseRear(1)+ell*cos(0.0);
                reverseRear(2)+ell*sin(0.0)];

    for k = 1:Np
        alpha = k/Np;
        Pref(:,k) = (1.0-alpha)*p0+alpha*reverseP;
        Uref(:,k) = [0.0;0.0];
    end

elseif mode == 6.0
    % Parked pose hold.
    goalP = [goalRear(1)+ell*cos(0.0);
             goalRear(2)+ell*sin(0.0)];

    for k = 1:Np
        Pref(:,k) = goalP;
        Uref(:,k) = [0.0;0.0];
    end

else
    % Timed trajMatrix tracking. In mode 5, refOffset was reset to the
    % first negative-v sample, so this follows the reverse-S segment from
    % its correct start.
    for k = 1:Np
        tq = tRef+k*Ts;

        [xr,yr,thr,vr,kr] = interpolateReference(ref,tq);

        cr = cos(thr);
        sr = sin(thr);

        Pref(:,k) = [xr+ell*cr;
                     yr+ell*sr];

        % Since theta_dot = v*kappa:
        % P_dot = v*e_theta + ell*v*kappa*e_perp
        Uref(:,k) = [vr*cr-ell*vr*kr*sr;
                     vr*sr+ell*vr*kr*cr];
    end
end

%% Quadratic MPC cost
H = 1e-6*eye(nz);
f = zeros(nz,1);

% Heavily penalized CBF slack. It prevents numerical infeasibility in the
% outer SCP. The inner safety filter should remain the hard safety layer.
H(nz,nz) = 2.0e6;

for k = 1:Np
    % P_k = p0 + S_k*z, where S acts only on the input part of z.
    S = zeros(2,nz);

    for j = 1:k
        cols = (2*j-1):(2*j);
        S(:,cols) = Ts*eye(2);
    end

    if k == Np
        Qk = Qf;
    else
        Qk = Q;
    end

    e0 = p0-Pref(:,k);

    H = H+2.0*(S.'*Qk*S);
    f = f+2.0*(S.'*Qk*e0);

    cols = (2*k-1):(2*k);
    H(cols,cols) = H(cols,cols)+2.0*R;
    f(cols)      = f(cols)-2.0*R*Uref(:,k);
end

% Smoothness with respect to the previously applied command.
idx0 = 1:2;
H(idx0,idx0) = H(idx0,idx0)+2.0*rhoDu*eye(2);
f(idx0)      = f(idx0)-2.0*rhoDu*uPrev;

% Smoothness between adjacent horizon commands.
for j = 2:Np
    im1 = (2*j-3):(2*j-2);
    i0  = (2*j-1):(2*j);

    H(im1,im1) = H(im1,im1)+2.0*rhoDu*eye(2);
    H(i0,i0)   = H(i0,i0)+2.0*rhoDu*eye(2);
    H(im1,i0)  = H(im1,i0)-2.0*rhoDu*eye(2);
    H(i0,im1)  = H(i0,im1)-2.0*rhoDu*eye(2);
end

H = 0.5*(H+H.');

%% Initial SCP rollout
zGuess = zWarm;
Pbar   = rolloutIntegrator(p0,zGuess,Ts,Np);

nCbfRows = Np*nObs;
A = zeros(nCbfRows,nz);
b = zeros(nCbfRows,1);

baseLB = -uMax*ones(nz,1);
baseUB =  uMax*ones(nz,1);

% CBF slack bounds.
baseLB(nz) = 0.0;
baseUB(nz) = 100.0;

lastGoodFlag = 0.0;
passes       = 0.0;
lastFlag     = -100.0;

qpOptions = optimoptions('quadprog', ...
    'Algorithm','interior-point-convex','Display','off');

%% Sequential convexification of the DCBF constraints
for scp = 1:nSCP
    A(:) = 0.0;
    b(:) = 0.0;
    row  = 0;

    for k = 1:Np
        % P_{k+1} = p0 + S*z.
        S = zeros(2,nz);

        for j = 1:k
            cols = (2*j-1):(2*j);
            S(:,cols) = Ts*eye(2);
        end

        for j = 1:nObs
            cObs = obs(j,1:2).';
            rObs = obs(j,3);

            pkBar    = Pbar(:,k);
            pNextBar = Pbar(:,k+1);

            dk    = pkBar-cObs;
            dNext = pNextBar-cObs;

            hK       = dk.'*dk-rObs*rObs;
            hNextBar = dNext.'*dNext-rObs*rObs;
            g        = 2.0*dNext;

            row = row+1;

            % hNextBar + g'*(P_{k+1}-pNextBar)
            %     >= (1-gamma)*hK - slack
            %
            % P_{k+1}=p0+S*z. Rewrite as A*z <= b.
            A(row,1:nInputs) = -(g.'*S(:,1:nInputs));
            A(row,nz)        = -1.0;

            b(row) = hNextBar ...
                     -g.'*pNextBar ...
                     +g.'*p0 ...
                     -(1.0-gammaCBF)*hK;
        end
    end

    lb = baseLB;
    ub = baseUB;

    if scp > 1
        lb(1:nInputs) = max(baseLB(1:nInputs), ...
                            zGuess(1:nInputs)-scpTrust);
        ub(1:nInputs) = min(baseUB(1:nInputs), ...
                            zGuess(1:nInputs)+scpTrust);
    end

    % quadprog returns an empty vector when it declares the QP infeasible.
    % Use a variable-size raw output and check its length before copying.
    zRaw = zeros(0,1);
    coder.varsize('zRaw',[nz 1],[true false]);
    flag = 0.0;

    [zRaw,~,flag] = quadprog( ...
        sparse(H),f,sparse(A),b,[],[],lb,ub,[],qpOptions);

    if flag > 0 && size(zRaw,1) == nz
        zCandidate = zRaw(1:nz);

        candidateOK = true;
        for i = 1:nz
            if ~isfinite(zCandidate(i))
                candidateOK = false;
            end
        end

        if candidateOK
            zGuess       = zCandidate;
            Pbar         = rolloutIntegrator(p0,zGuess,Ts,Np);
            passes       = scp;
            lastGoodFlag = flag;
        else
            lastFlag = flag;
            break;
        end
    else
        lastFlag = flag;
        break;
    end
end

if passes == 0
    % Safe fallback for stationary obstacles and an initially safe P.
    zGuess = zeros(nz,1);
    Pbar   = rolloutIntegrator(p0,zGuess,Ts,Np);
    qp_status = lastFlag;
else
    qp_status = lastGoodFlag;
end

%% Outputs and warm-start update
u1_cmd = zGuess(1);
u2_cmd = zGuess(2);

P_pred_out     = Pbar;
scp_passes_out = passes;

% Shift the virtual-input solution by one sampling interval.
zNextWarm = zeros(nz,1);
zNextWarm(1:nInputs-2) = zGuess(3:nInputs);
zNextWarm(nInputs-1:nInputs) = zGuess(nInputs-1:nInputs);
zNextWarm(nz) = 0.0;

zWarm = zNextWarm;
uPrev = zGuess(1:2);
tPrev = t;

end

%% -----------------------------------------------------------------------
function P = rolloutIntegrator(p0,z,Ts,Np)

P = zeros(2,Np+1);
P(:,1) = p0;

for k = 1:Np
    cols = (2*k-1):(2*k);
    P(:,k+1) = P(:,k)+Ts*z(cols);
end

end

%% -----------------------------------------------------------------------
function hMin = obstacle3Barrier(x,cx,cy,r,L)

th = x(3);

rearD = [x(1)-cx;
         x(2)-cy];

frontD = [x(1)+L*cos(th)-cx;
          x(2)+L*sin(th)-cy];

hRear  = rearD.'*rearD-r*r;
hFront = frontD.'*frontD-r*r;
hMin   = min(hRear,hFront);

end


%% -----------------------------------------------------------------------
function tReverse = findReverseStartTime(ref)

n = size(ref,1);
nValid = 1;

for i = 2:n
    if ref(i,1) > ref(i-1,1)+1e-9
        nValid = i;
    else
        break;
    end
end

tReverse = ref(nValid,1);

for i = 1:nValid
    if ref(i,5) < -1e-6
        tReverse = ref(i,1);
        return;
    end
end

end

%% -----------------------------------------------------------------------
function [xr,yr,thr,vr,kr] = interpolateReference(ref,tq)

n = size(ref,1);
nValid = 1;

for i = 2:n
    if ref(i,1) > ref(i-1,1)+1e-9
        nValid = i;
    else
        break;
    end
end

if tq <= ref(1,1)
    xr  = ref(1,2);
    yr  = ref(1,3);
    thr = ref(1,4);
    vr  = ref(1,5);
    kr  = ref(1,6);
    return;
end

if tq >= ref(nValid,1)
    xr  = ref(nValid,2);
    yr  = ref(nValid,3);
    thr = ref(nValid,4);
    vr  = ref(nValid,5);
    kr  = ref(nValid,6);
    return;
end

idx = 1;

while idx < nValid-1 && ref(idx+1,1) < tq
    idx = idx+1;
end

t0 = ref(idx,1);
t1 = ref(idx+1,1);

if t1 > t0
    alpha = (tq-t0)/(t1-t0);
else
    alpha = 0.0;
end

alpha = max(0.0,min(1.0,alpha));

xr  = (1-alpha)*ref(idx,2)+alpha*ref(idx+1,2);
yr  = (1-alpha)*ref(idx,3)+alpha*ref(idx+1,3);
thr = (1-alpha)*ref(idx,4)+alpha*ref(idx+1,4);
vr  = (1-alpha)*ref(idx,5)+alpha*ref(idx+1,5);
kr  = (1-alpha)*ref(idx,6)+alpha*ref(idx+1,6);

end

%% -----------------------------------------------------------------------
function tAtX = findReferenceTimeAtX(ref,xQuery)
% Used only on the forward part of the trajectory, where x is monotonic.

n = size(ref,1);
nValid = 1;

for i = 2:n
    if ref(i,1) > ref(i-1,1)+1e-9
        nValid = i;
    else
        break;
    end
end

tAtX = ref(nValid,1);

for i = 1:nValid
    if ref(i,2) >= xQuery
        tAtX = ref(i,1);
        return;
    end
end

end

== matlab function MPC_FL_CBFcontroller/Robot Bicycle Model/wrapToPi ==
  data: qIn input; qOut output
function qOut = wrapToPi(qIn)
%#codegen

qOut = angdiff(0*qIn, qIn);
